simulink model "tongbukongzhi1"  (R2014b)
settings: Solver=ode45  StartTime=0.0  StopTime=10.0  RelTol=1e-3
undefined symbols (not defined in the file): sigbuilder_block
libraries: simulink x61, fuzblock x32
(part 4 of 4)

== system tongbukongzhi1/Subsystem1/Subsystem5/fuzzypid2/Subsystem ==
  In1 : Inport
  In2 : Inport  Port=2
  Add : Sum  Inputs=+++
  Demux : Demux  Outputs=3
  Derivative : Derivative
  Fuzzy Logic Controller : fuzblock/Fuzzy Logic  Controller  fis=fuzzy1
  Gain : Gain  Gain=12.9851074749726
  Gain1 : Gain  Gain=3.96505413373294
  Gain2 : Gain  Gain=0.756963167778154
  Integrator : Integrator
  Mux : Mux  Inputs=2
  Mux1 : Mux  Inputs=3
  Scope : Scope
  Sum : Sum  Inputs=|++
  Sum1 : Sum  Inputs=|++
  Sum2 : Sum  Inputs=|++
  Zero-Order Hold : ZeroOrderHold  SampleTime=0.2
  Zero-Order Hold1 : ZeroOrderHold  SampleTime=0.2
  Out1 : Outport
  wires:
  In1/1 -> Gain/1, Gain2/1, Gain1/1, Mux/1
  Derivative/1 -> Add/3
  Integrator/1 -> Add/2
  Add/1 -> Out1/1
  In2/1 -> Mux/2
  Gain/1 -> Sum2/1
  Sum2/1 -> Add/1
  Gain1/1 -> Sum1/1
  Sum1/1 -> Integrator/1
  Gain2/1 -> Sum/1
  Sum/1 -> Derivative/1
  Demux/1 -> Mux1/1, Sum2/2
  Demux/2 -> Sum1/2, Mux1/2
  Demux/3 -> Sum/2, Mux1/3
  Mux/1 -> Zero-Order Hold/1
  Fuzzy Logic Controller/1 -> Zero-Order Hold1/1
  Zero-Order Hold/1 -> Fuzzy Logic Controller/1
  Zero-Order Hold1/1 -> Demux/1
  Mux1/1 -> Scope/1

== system tongbukongzhi1/Subsystem1/Subsystem5/fuzzypid3/Subsystem ==
  In1 : Inport
  In2 : Inport  Port=2
  Add : Sum  Inputs=+++
  Demux : Demux  Outputs=3
  Derivative : Derivative
  Fuzzy Logic Controller : fuzblock/Fuzzy Logic  Controller  fis=fuzzy1
  Gain : Gain  Gain=12.9851074749726
  Gain1 : Gain  Gain=3.96505413373294
  Gain2 : Gain  Gain=0.756963167778154
  Integrator : Integrator
  Mux : Mux  Inputs=2
  Mux1 : Mux  Inputs=3
  Scope : Scope
  Sum : Sum  Inputs=|++
  Sum1 : Sum  Inputs=|++
  Sum2 : Sum  Inputs=|++
  Zero-Order Hold : ZeroOrderHold  SampleTime=0.2
  Zero-Order Hold1 : ZeroOrderHold  SampleTime=0.2
  Out1 : Outport
  wires:
  In1/1 -> Gain/1, Gain2/1, Gain1/1, Mux/1
  Derivative/1 -> Add/3
  Integrator/1 -> Add/2
  Add/1 -> Out1/1
  In2/1 -> Mux/2
  Gain/1 -> Sum2/1
  Sum2/1 -> Add/1
  Gain1/1 -> Sum1/1
  Sum1/1 -> Integrator/1
  Gain2/1 -> Sum/1
  Sum/1 -> Derivative/1
  Demux/1 -> Mux1/1, Sum2/2
  Demux/2 -> Sum1/2, Mux1/2
  Demux/3 -> Sum/2, Mux1/3
  Mux/1 -> Zero-Order Hold/1
  Fuzzy Logic Controller/1 -> Zero-Order Hold1/1
  Zero-Order Hold/1 -> Fuzzy Logic Controller/1
  Zero-Order Hold1/1 -> Demux/1
  Mux1/1 -> Scope/1

== system tongbukongzhi1/Subsystem1/Subsystem6/fuzzypid1/Subsystem ==
  In1 : Inport
  In2 : Inport  Port=2
  Add : Sum  Inputs=+++
  Demux : Demux  Outputs=3
  Derivative : Derivative
  Fuzzy Logic Controller : fuzblock/Fuzzy Logic  Controller  fis=fuzzy1
  Gain : Gain  Gain=12.9851074749726
  Gain1 : Gain  Gain=3.96505413373294
  Gain2 : Gain  Gain=0.756963167778154
  Integrator : Integrator
  Mux : Mux  Inputs=2
  Mux1 : Mux  Inputs=3
  Scope : Scope
  Sum : Sum  Inputs=|++
  Sum1 : Sum  Inputs=|++
  Sum2 : Sum  Inputs=|++
  Zero-Order Hold : ZeroOrderHold  SampleTime=0.2
  Zero-Order Hold1 : ZeroOrderHold  SampleTime=0.2
  Out1 : Outport
  wires:
  In1/1 -> Gain/1, Gain2/1, Gain1/1, Mux/1
  Derivative/1 -> Add/3
  Integrator/1 -> Add/2
  Add/1 -> Out1/1
  In2/1 -> Mux/2
  Gain/1 -> Sum2/1
  Sum2/1 -> Add/1
  Gain1/1 -> Sum1/1
  Sum1/1 -> Integrator/1
  Gain2/1 -> Sum/1
  Sum/1 -> Derivative/1
  Demux/1 -> Mux1/1, Sum2/2
  Demux/2 -> Sum1/2, Mux1/2
  Demux/3 -> Sum/2, Mux1/3
  Mux/1 -> Zero-Order Hold/1
  Fuzzy Logic Controller/1 -> Zero-Order Hold1/1
  Zero-Order Hold/1 -> Fuzzy Logic Controller/1
  Zero-Order Hold1/1 -> Demux/1
  Mux1/1 -> Scope/1

== system tongbukongzhi1/Subsystem1/Subsystem6/fuzzypid2/Subsystem ==
  In1 : Inport
  In2 : Inport  Port=2
  Add : Sum  Inputs=+++
  Demux : Demux  Outputs=3
  Derivative : Derivative
  Fuzzy Logic Controller : fuzblock/Fuzzy Logic  Controller  fis=fuzzy1
  Gain : Gain  Gain=12.9851074749726
  Gain1 : Gain  Gain=3.96505413373294
  Gain2 : Gain  Gain=0.756963167778154
  Integrator : Integrator
  Mux : Mux  Inputs=2
  Mux1 : Mux  Inputs=3
  Scope : Scope
  Sum : Sum  Inputs=|++
  Sum1 : Sum  Inputs=|++
  Sum2 : Sum  Inputs=|++
  Zero-Order Hold : ZeroOrderHold  SampleTime=0.2
  Zero-Order Hold1 : ZeroOrderHold  SampleTime=0.2
  Out1 : Outport
  wires:
  In1/1 -> Gain/1, Gain2/1, Gain1/1, Mux/1
  Derivative/1 -> Add/3
  Integrator/1 -> Add/2
  Add/1 -> Out1/1
  In2/1 -> Mux/2
  Gain/1 -> Sum2/1
  Sum2/1 -> Add/1
  Gain1/1 -> Sum1/1
  Sum1/1 -> Integrator/1
  Gain2/1 -> Sum/1
  Sum/1 -> Derivative/1
  Demux/1 -> Mux1/1, Sum2/2
  Demux/2 -> Sum1/2, Mux1/2
  Demux/3 -> Sum/2, Mux1/3
  Mux/1 -> Zero-Order Hold/1
  Fuzzy Logic Controller/1 -> Zero-Order Hold1/1
  Zero-Order Hold/1 -> Fuzzy Logic Controller/1
  Zero-Order Hold1/1 -> Demux/1
  Mux1/1 -> Scope/1

== system tongbukongzhi1/Subsystem1/Subsystem6/fuzzypid3/Subsystem ==
  In1 : Inport
  In2 : Inport  Port=2
  Add : Sum  Inputs=+++
  Demux : Demux  Outputs=3
  Derivative : Derivative
  Fuzzy Logic Controller : fuzblock/Fuzzy Logic  Controller  fis=fuzzy1
  Gain : Gain  Gain=12.9851074749726
  Gain1 : Gain  Gain=3.96505413373294
  Gain2 : Gain  Gain=0.756963167778154
  Integrator : Integrator
  Mux : Mux  Inputs=2
  Mux1 : Mux  Inputs=3
  Scope : Scope
  Sum : Sum  Inputs=|++
  Sum1 : Sum  Inputs=|++
  Sum2 : Sum  Inputs=|++
  Zero-Order Hold : ZeroOrderHold  SampleTime=0.2
  Zero-Order Hold1 : ZeroOrderHold  SampleTime=0.2
  Out1 : Outport
  wires:
  In1/1 -> Gain/1, Gain2/1, Gain1/1, Mux/1
  Derivative/1 -> Add/3
  Integrator/1 -> Add/2
  Add/1 -> Out1/1
  In2/1 -> Mux/2
  Gain/1 -> Sum2/1
  Sum2/1 -> Add/1
  Gain1/1 -> Sum1/1
  Sum1/1 -> Integrator/1
  Gain2/1 -> Sum/1
  Sum/1 -> Derivative/1
  Demux/1 -> Mux1/1, Sum2/2
  Demux/2 -> Sum1/2, Mux1/2
  Demux/3 -> Sum/2, Mux1/3
  Mux/1 -> Zero-Order Hold/1
  Fuzzy Logic Controller/1 -> Zero-Order Hold1/1
  Zero-Order Hold/1 -> Fuzzy Logic Controller/1
  Zero-Order Hold1/1 -> Demux/1
  Mux1/1 -> Scope/1

== system tongbukongzhi1/Subsystem1/Subsystem7/fuzzypid1/Subsystem ==
  In1 : Inport
  In2 : Inport  Port=2
  Add : Sum  Inputs=+++
  Demux : Demux  Outputs=3
  Derivative : Derivative
  Fuzzy Logic Controller : fuzblock/Fuzzy Logic  Controller  fis=fuzzy1
  Gain : Gain  Gain=12.9851074749726
  Gain1 : Gain  Gain=3.96505413373294
  Gain2 : Gain  Gain=0.756963167778154
  Integrator : Integrator
  Mux : Mux  Inputs=2
  Mux1 : Mux  Inputs=3
  Scope : Scope
  Sum : Sum  Inputs=|++
  Sum1 : Sum  Inputs=|++
  Sum2 : Sum  Inputs=|++
  Zero-Order Hold : ZeroOrderHold  SampleTime=0.2
  Zero-Order Hold1 : ZeroOrderHold  SampleTime=0.2
  Out1 : Outport
  wires:
  In1/1 -> Gain/1, Gain2/1, Gain1/1, Mux/1
  Derivative/1 -> Add/3
  Integrator/1 -> Add/2
  Add/1 -> Out1/1
  In2/1 -> Mux/2
  Gain/1 -> Sum2/1
  Sum2/1 -> Add/1
  Gain1/1 -> Sum1/1
  Sum1/1 -> Integrator/1
  Gain2/1 -> Sum/1
  Sum/1 -> Derivative/1
  Demux/1 -> Mux1/1, Sum2/2
  Demux/2 -> Sum1/2, Mux1/2
  Demux/3 -> Sum/2, Mux1/3
  Mux/1 -> Zero-Order Hold/1
  Fuzzy Logic Controller/1 -> Zero-Order Hold1/1
  Zero-Order Hold/1 -> Fuzzy Logic Controller/1
  Zero-Order Hold1/1 -> Demux/1
  Mux1/1 -> Scope/1

== system tongbukongzhi1/Subsystem1/Subsystem7/fuzzypid2/Subsystem ==
  In1 : Inport
  In2 : Inport  Port=2
  Add : Sum  Inputs=+++
  Demux : Demux  Outputs=3
  Derivative : Derivative
  Fuzzy Logic Controller : fuzblock/Fuzzy Logic  Controller  fis=fuzzy1
  Gain : Gain  Gain=12.9851074749726
  Gain1 : Gain  Gain=3.96505413373294
  Gain2 : Gain  Gain=0.756963167778154
  Integrator : Integrator
  Mux : Mux  Inputs=2
  Mux1 : Mux  Inputs=3
  Scope : Scope
  Sum : Sum  Inputs=|++
  Sum1 : Sum  Inputs=|++
  Sum2 : Sum  Inputs=|++
  Zero-Order Hold : ZeroOrderHold  SampleTime=0.2
  Zero-Order Hold1 : ZeroOrderHold  SampleTime=0.2
  Out1 : Outport
  wires:
  In1/1 -> Gain/1, Gain2/1, Gain1/1, Mux/1
  Derivative/1 -> Add/3
  Integrator/1 -> Add/2
  Add/1 -> Out1/1
  In2/1 -> Mux/2
  Gain/1 -> Sum2/1
  Sum2/1 -> Add/1
  Gain1/1 -> Sum1/1
  Sum1/1 -> Integrator/1
  Gain2/1 -> Sum/1
  Sum/1 -> Derivative/1
  Demux/1 -> Mux1/1, Sum2/2
  Demux/2 -> Sum1/2, Mux1/2
  Demux/3 -> Sum/2, Mux1/3
  Mux/1 -> Zero-Order Hold/1
  Fuzzy Logic Controller/1 -> Zero-Order Hold1/1
  Zero-Order Hold/1 -> Fuzzy Logic Controller/1
  Zero-Order Hold1/1 -> Demux/1
  Mux1/1 -> Scope/1

== system tongbukongzhi1/Subsystem1/Subsystem7/fuzzypid3/Subsystem ==
  In1 : Inport
  In2 : Inport  Port=2
  Add : Sum  Inputs=+++
  Demux : Demux  Outputs=3
  Derivative : Derivative
  Fuzzy Logic Controller : fuzblock/Fuzzy Logic  Controller  fis=fuzzy1
  Gain : Gain  Gain=12.9851074749726
  Gain1 : Gain  Gain=3.96505413373294
  Gain2 : Gain  Gain=0.756963167778154
  Integrator : Integrator
  Mux : Mux  Inputs=2
  Mux1 : Mux  Inputs=3
  Scope : Scope
  Sum : Sum  Inputs=|++
  Sum1 : Sum  Inputs=|++
  Sum2 : Sum  Inputs=|++
  Zero-Order Hold : ZeroOrderHold  SampleTime=0.2
  Zero-Order Hold1 : ZeroOrderHold  SampleTime=0.2
  Out1 : Outport
  wires:
  In1/1 -> Gain/1, Gain2/1, Gain1/1, Mux/1
  Derivative/1 -> Add/3
  Integrator/1 -> Add/2
  Add/1 -> Out1/1
  In2/1 -> Mux/2
  Gain/1 -> Sum2/1
  Sum2/1 -> Add/1
  Gain1/1 -> Sum1/1
  Sum1/1 -> Integrator/1
  Gain2/1 -> Sum/1
  Sum/1 -> Derivative/1
  Demux/1 -> Mux1/1, Sum2/2
  Demux/2 -> Sum1/2, Mux1/2
  Demux/3 -> Sum/2, Mux1/3
  Mux/1 -> Zero-Order Hold/1
  Fuzzy Logic Controller/1 -> Zero-Order Hold1/1
  Zero-Order Hold/1 -> Fuzzy Logic Controller/1
  Zero-Order Hold1/1 -> Demux/1
  Mux1/1 -> Scope/1

== system tongbukongzhi1/Subsystem4/Subsystem/fuzzypid1/Subsystem ==
  In1 : Inport
  In2 : Inport  Port=2
  Add : Sum  Inputs=+++
  Demux : Demux  Outputs=3
  Derivative : Derivative
  Fuzzy Logic Controller : fuzblock/Fuzzy Logic  Controller  fis=fuzzy1
  Gain : Gain  Gain=12.9851074749726
  Gain1 : Gain  Gain=3.96505413373294
  Gain2 : Gain  Gain=0.756963167778154
  Integrator : Integrator
  Mux : Mux  Inputs=2
  Mux1 : Mux  Inputs=3
  Scope : Scope
      settings: YMin=-0.2  YMax=0.05
  Sum : Sum  Inputs=|++
  Sum1 : Sum  Inputs=|++
  Sum2 : Sum  Inputs=|++
  Zero-Order Hold : ZeroOrderHold  SampleTime=0.1
  Zero-Order Hold1 : ZeroOrderHold  SampleTime=0.1
  Out1 : Outport
  wires:
  In1/1 -> Gain/1, Gain2/1, Gain1/1, Mux/1
  Derivative/1 -> Add/3
  Integrator/1 -> Add/2
  Add/1 -> Out1/1
  In2/1 -> Mux/2
  Gain/1 -> Sum2/1
  Sum2/1 -> Add/1
  Gain1/1 -> Sum1/1
  Sum1/1 -> Integrator/1
  Gain2/1 -> Sum/1
  Sum/1 -> Derivative/1
  Mux/1 -> Zero-Order Hold/1
  Fuzzy Logic Controller/1 -> Zero-Order Hold1/1
  Zero-Order Hold/1 -> Fuzzy Logic Controller/1
  Zero-Order Hold1/1 -> Demux/1
  Mux1/1 -> Scope/1
  Demux/3 -> Sum/2, Mux1/3
  Demux/2 -> Sum1/2, Mux1/2
  Demux/1 -> Mux1/1, Sum2/2

== system tongbukongzhi1/Subsystem4/Subsystem/fuzzypid2/Subsystem ==
  In1 : Inport
  In2 : Inport  Port=2
  Add : Sum  Inputs=+++
  Demux : Demux  Outputs=3
  Derivative : Derivative
  Fuzzy Logic Controller : fuzblock/Fuzzy Logic  Controller  fis=fuzzy1
  Gain : Gain  Gain=12.9851074749726
  Gain1 : Gain  Gain=3.96505413373294
  Gain2 : Gain  Gain=0.756963167778154
  Integrator : Integrator
  Mux : Mux  Inputs=2
  Mux1 : Mux  Inputs=3
  Scope : Scope
      settings: YMin=-0.2  YMax=0.05
  Sum : Sum  Inputs=|++
  Sum1 : Sum  Inputs=|++
  Sum2 : Sum  Inputs=|++
  Zero-Order Hold : ZeroOrderHold  SampleTime=0.1
  Zero-Order Hold1 : ZeroOrderHold  SampleTime=0.1
  Out1 : Outport
  wires:
  In1/1 -> Gain/1, Gain2/1, Gain1/1, Mux/1
  Derivative/1 -> Add/3
  Integrator/1 -> Add/2
  Add/1 -> Out1/1
  In2/1 -> Mux/2
  Gain/1 -> Sum2/1
  Sum2/1 -> Add/1
  Gain1/1 -> Sum1/1
  Sum1/1 -> Integrator/1
  Gain2/1 -> Sum/1
  Sum/1 -> Derivative/1
  Mux/1 -> Zero-Order Hold/1
  Fuzzy Logic Controller/1 -> Zero-Order Hold1/1
  Zero-Order Hold/1 -> Fuzzy Logic Controller/1
  Zero-Order Hold1/1 -> Demux/1
  Mux1/1 -> Scope/1
  Demux/3 -> Sum/2, Mux1/3
  Demux/2 -> Sum1/2, Mux1/2
  Demux/1 -> Mux1/1, Sum2/2

== system tongbukongzhi1/Subsystem4/Subsystem/fuzzypid4/Subsystem ==
  In1 : Inport
  In2 : Inport  Port=2
  Add : Sum  Inputs=+++
  Demux : Demux  Outputs=3
  Derivative : Derivative
  Fuzzy Logic Controller : fuzblock/Fuzzy Logic  Controller  fis=fuzzy1
  Gain : Gain  Gain=12.9851074749726
  Gain1 : Gain  Gain=3.96505413373294
  Gain2 : Gain  Gain=0.756963167778154
  Integrator : Integrator
  Mux : Mux  Inputs=2
  Mux1 : Mux  Inputs=3
  Scope : Scope
      settings: YMin=-0.2  YMax=0.05
  Sum : Sum  Inputs=|++
  Sum1 : Sum  Inputs=|++
  Sum2 : Sum  Inputs=|++
  Zero-Order Hold : ZeroOrderHold  SampleTime=0.1
  Zero-Order Hold1 : ZeroOrderHold  SampleTime=0.1
  Out1 : Outport
  wires:
  In1/1 -> Gain/1, Gain2/1, Gain1/1, Mux/1
  Derivative/1 -> Add/3
  Integrator/1 -> Add/2
  Add/1 -> Out1/1
  In2/1 -> Mux/2
  Gain/1 -> Sum2/1
  Sum2/1 -> Add/1
  Gain1/1 -> Sum1/1
  Sum1/1 -> Integrator/1
  Gain2/1 -> Sum/1
  Sum/1 -> Derivative/1
  Mux/1 -> Zero-Order Hold/1
  Fuzzy Logic Controller/1 -> Zero-Order Hold1/1
  Zero-Order Hold/1 -> Fuzzy Logic Controller/1
  Zero-Order Hold1/1 -> Demux/1
  Mux1/1 -> Scope/1
  Demux/3 -> Sum/2, Mux1/3
  Demux/2 -> Sum1/2, Mux1/2
  Demux/1 -> Mux1/1, Sum2/2

== system tongbukongzhi1/Subsystem4/Subsystem1/fuzzypid4/Subsystem ==
  In1 : Inport
  In2 : Inport  Port=2
  Add : Sum  Inputs=+++
  Demux : Demux  Outputs=3
  Derivative : Derivative
  Fuzzy Logic Controller : fuzblock/Fuzzy Logic  Controller  fis=fuzzy1
  Gain : Gain  Gain=12.9851074749726
  Gain1 : Gain  Gain=3.96505413373294
  Gain2 : Gain  Gain=0.756963167778154
  Integrator : Integrator
  Mux : Mux  Inputs=2
  Mux1 : Mux  Inputs=3
  Scope : Scope
      settings: YMin=-0.2  YMax=0.05
  Sum : Sum  Inputs=|++
  Sum1 : Sum  Inputs=|++
  Sum2 : Sum  Inputs=|++
  Zero-Order Hold : ZeroOrderHold  SampleTime=0.1
  Zero-Order Hold1 : ZeroOrderHold  SampleTime=0.1
  Out1 : Outport
  wires:
  In1/1 -> Gain/1, Gain2/1, Gain1/1, Mux/1
  Derivative/1 -> Add/3
  Integrator/1 -> Add/2
  Add/1 -> Out1/1
  In2/1 -> Mux/2
  Gain/1 -> Sum2/1
  Sum2/1 -> Add/1
  Gain1/1 -> Sum1/1
  Sum1/1 -> Integrator/1
  Gain2/1 -> Sum/1
  Sum/1 -> Derivative/1
  Mux/1 -> Zero-Order Hold/1
  Fuzzy Logic Controller/1 -> Zero-Order Hold1/1
  Zero-Order Hold/1 -> Fuzzy Logic Controller/1
  Zero-Order Hold1/1 -> Demux/1
  Mux1/1 -> Scope/1
  Demux/3 -> Sum/2, Mux1/3
  Demux/2 -> Sum1/2, Mux1/2
  Demux/1 -> Mux1/1, Sum2/2

== system tongbukongzhi1/Subsystem4/Subsystem1/fuzzypid5/Subsystem ==
  In1 : Inport
  In2 : Inport  Port=2
  Add : Sum  Inputs=+++
  Demux : Demux  Outputs=3
  Derivative : Derivative
  Fuzzy Logic Controller : fuzblock/Fuzzy Logic  Controller  fis=fuzzy1
  Gain : Gain  Gain=12.9851074749726
  Gain1 : Gain  Gain=3.96505413373294
  Gain2 : Gain  Gain=0.756963167778154
  Integrator : Integrator
  Mux : Mux  Inputs=2
  Mux1 : Mux  Inputs=3
  Scope : Scope
      settings: YMin=-0.2  YMax=0.05
  Sum : Sum  Inputs=|++
  Sum1 : Sum  Inputs=|++
  Sum2 : Sum  Inputs=|++
  Zero-Order Hold : ZeroOrderHold  SampleTime=0.1
  Zero-Order Hold1 : ZeroOrderHold  SampleTime=0.1
  Out1 : Outport
  wires:
  In1/1 -> Gain/1, Gain2/1, Gain1/1, Mux/1
  Derivative/1 -> Add/3
  Integrator/1 -> Add/2
  Add/1 -> Out1/1
  In2/1 -> Mux/2
  Gain/1 -> Sum2/1
  Sum2/1 -> Add/1
  Gain1/1 -> Sum1/1
  Sum1/1 -> Integrator/1
  Gain2/1 -> Sum/1
  Sum/1 -> Derivative/1
  Mux/1 -> Zero-Order Hold/1
  Fuzzy Logic Controller/1 -> Zero-Order Hold1/1
  Zero-Order Hold/1 -> Fuzzy Logic Controller/1
  Zero-Order Hold1/1 -> Demux/1
  Mux1/1 -> Scope/1
  Demux/3 -> Sum/2, Mux1/3
  Demux/2 -> Sum1/2, Mux1/2
  Demux/1 -> Mux1/1, Sum2/2

== system tongbukongzhi1/Subsystem4/Subsystem1/fuzzypid6/Subsystem ==
  In1 : Inport
  In2 : Inport  Port=2
  Add : Sum  Inputs=+++
  Demux : Demux  Outputs=3
  Derivative : Derivative
  Fuzzy Logic Controller : fuzblock/Fuzzy Logic  Controller  fis=fuzzy1
  Gain : Gain  Gain=12.9851074749726
  Gain1 : Gain  Gain=3.96505413373294
  Gain2 : Gain  Gain=0.756963167778154
  Integrator : Integrator
  Mux : Mux  Inputs=2
  Mux1 : Mux  Inputs=3
  Scope : Scope
      settings: YMin=-0.2  YMax=0.05
  Sum : Sum  Inputs=|++
  Sum1 : Sum  Inputs=|++
  Sum2 : Sum  Inputs=|++
  Zero-Order Hold : ZeroOrderHold  SampleTime=0.1
  Zero-Order Hold1 : ZeroOrderHold  SampleTime=0.1
  Out1 : Outport
  wires:
  In1/1 -> Gain/1, Gain2/1, Gain1/1, Mux/1
  Derivative/1 -> Add/3
  Integrator/1 -> Add/2
  Add/1 -> Out1/1
  In2/1 -> Mux/2
  Gain/1 -> Sum2/1
  Sum2/1 -> Add/1
  Gain1/1 -> Sum1/1
  Sum1/1 -> Integrator/1
  Gain2/1 -> Sum/1
  Sum/1 -> Derivative/1
  Mux/1 -> Zero-Order Hold/1
  Fuzzy Logic Controller/1 -> Zero-Order Hold1/1
  Zero-Order Hold/1 -> Fuzzy Logic Controller/1
  Zero-Order Hold1/1 -> Demux/1
  Mux1/1 -> Scope/1
  Demux/3 -> Sum/2, Mux1/3
  Demux/2 -> Sum1/2, Mux1/2
  Demux/1 -> Mux1/1, Sum2/2

== system tongbukongzhi1/Subsystem4/Subsystem2/fuzzypid4/Subsystem ==
  In1 : Inport
  In2 : Inport  Port=2
  Add : Sum  Inputs=+++
  Demux : Demux  Outputs=3
  Derivative : Derivative
  Fuzzy Logic Controller : fuzblock/Fuzzy Logic  Controller  fis=fuzzy1
  Gain : Gain  Gain=12.9851074749726
  Gain1 : Gain  Gain=3.96505413373294
  Gain2 : Gain  Gain=0.756963167778154
  Integrator : Integrator
  Mux : Mux  Inputs=2
  Mux1 : Mux  Inputs=3
  Scope : Scope
      settings: YMin=-0.2  YMax=0.05
  Sum : Sum  Inputs=|++
  Sum1 : Sum  Inputs=|++
  Sum2 : Sum  Inputs=|++
  Zero-Order Hold : ZeroOrderHold  SampleTime=0.1
  Zero-Order Hold1 : ZeroOrderHold  SampleTime=0.1
  Out1 : Outport
  wires:
  In1/1 -> Gain/1, Gain2/1, Gain1/1, Mux/1
  Derivative/1 -> Add/3
  Integrator/1 -> Add/2
  Add/1 -> Out1/1
  In2/1 -> Mux/2
  Gain/1 -> Sum2/1
  Sum2/1 -> Add/1
  Gain1/1 -> Sum1/1
  Sum1/1 -> Integrator/1
  Gain2/1 -> Sum/1
  Sum/1 -> Derivative/1
  Mux/1 -> Zero-Order Hold/1
  Fuzzy Logic Controller/1 -> Zero-Order Hold1/1
  Zero-Order Hold/1 -> Fuzzy Logic Controller/1
  Zero-Order Hold1/1 -> Demux/1
  Mux1/1 -> Scope/1
  Demux/3 -> Sum/2, Mux1/3
  Demux/2 -> Sum1/2, Mux1/2
  Demux/1 -> Mux1/1, Sum2/2

== system tongbukongzhi1/Subsystem4/Subsystem2/fuzzypid5/Subsystem ==
  In1 : Inport
  In2 : Inport  Port=2
  Add : Sum  Inputs=+++
  Demux : Demux  Outputs=3
  Derivative : Derivative
  Fuzzy Logic Controller : fuzblock/Fuzzy Logic  Controller  fis=fuzzy1
  Gain : Gain  Gain=12.9851074749726
  Gain1 : Gain  Gain=3.96505413373294
  Gain2 : Gain  Gain=0.756963167778154
  Integrator : Integrator
  Mux : Mux  Inputs=2
  Mux1 : Mux  Inputs=3
  Scope : Scope
      settings: YMin=-0.2  YMax=0.05
  Sum : Sum  Inputs=|++
  Sum1 : Sum  Inputs=|++
  Sum2 : Sum  Inputs=|++
  Zero-Order Hold : ZeroOrderHold  SampleTime=0.1
  Zero-Order Hold1 : ZeroOrderHold  SampleTime=0.1
  Out1 : Outport
  wires:
  In1/1 -> Gain/1, Gain2/1, Gain1/1, Mux/1
  Derivative/1 -> Add/3
  Integrator/1 -> Add/2
  Add/1 -> Out1/1
  In2/1 -> Mux/2
  Gain/1 -> Sum2/1
  Sum2/1 -> Add/1
  Gain1/1 -> Sum1/1
  Sum1/1 -> Integrator/1
  Gain2/1 -> Sum/1
  Sum/1 -> Derivative/1
  Mux/1 -> Zero-Order Hold/1
  Fuzzy Logic Controller/1 -> Zero-Order Hold1/1
  Zero-Order Hold/1 -> Fuzzy Logic Controller/1
  Zero-Order Hold1/1 -> Demux/1
  Mux1/1 -> Scope/1
  Demux/3 -> Sum/2, Mux1/3
  Demux/2 -> Sum1/2, Mux1/2
  Demux/1 -> Mux1/1, Sum2/2

== system tongbukongzhi1/Subsystem4/Subsystem2/fuzzypid6/Subsystem ==
  In1 : Inport
  In2 : Inport  Port=2
  Add : Sum  Inputs=+++
  Demux : Demux  Outputs=3
  Derivative : Derivative
  Fuzzy Logic Controller : fuzblock/Fuzzy Logic  Controller  fis=fuzzy1
  Gain : Gain  Gain=12.9851074749726
  Gain1 : Gain  Gain=3.96505413373294
  Gain2 : Gain  Gain=0.756963167778154
  Integrator : Integrator
  Mux : Mux  Inputs=2
  Mux1 : Mux  Inputs=3
  Scope : Scope
      settings: YMin=-0.2  YMax=0.05
  Sum : Sum  Inputs=|++
  Sum1 : Sum  Inputs=|++
  Sum2 : Sum  Inputs=|++
  Zero-Order Hold : ZeroOrderHold  SampleTime=0.1
  Zero-Order Hold1 : ZeroOrderHold  SampleTime=0.1
  Out1 : Outport
  wires:
  In1/1 -> Gain/1, Gain2/1, Gain1/1, Mux/1
  Derivative/1 -> Add/3
  Integrator/1 -> Add/2
  Add/1 -> Out1/1
  In2/1 -> Mux/2
  Gain/1 -> Sum2/1
  Sum2/1 -> Add/1
  Gain1/1 -> Sum1/1
  Sum1/1 -> Integrator/1
  Gain2/1 -> Sum/1
  Sum/1 -> Derivative/1
  Mux/1 -> Zero-Order Hold/1
  Fuzzy Logic Controller/1 -> Zero-Order Hold1/1
  Zero-Order Hold/1 -> Fuzzy Logic Controller/1
  Zero-Order Hold1/1 -> Demux/1
  Mux1/1 -> Scope/1
  Demux/3 -> Sum/2, Mux1/3
  Demux/2 -> Sum1/2, Mux1/2
  Demux/1 -> Mux1/1, Sum2/2

== system tongbukongzhi1/Subsystem4/Subsystem3/fuzzypid4/Subsystem ==
  In1 : Inport
  In2 : Inport  Port=2
  Add : Sum  Inputs=+++
  Demux : Demux  Outputs=3
  Derivative : Derivative
  Fuzzy Logic Controller : fuzblock/Fuzzy Logic  Controller  fis=fuzzy1
  Gain : Gain  Gain=12.9851074749726
  Gain1 : Gain  Gain=3.96505413373294
  Gain2 : Gain  Gain=0.756963167778154
  Integrator : Integrator
  Mux : Mux  Inputs=2
  Mux1 : Mux  Inputs=3
  Scope : Scope
      settings: YMin=-0.2  YMax=0.05
  Sum : Sum  Inputs=|++
  Sum1 : Sum  Inputs=|++
  Sum2 : Sum  Inputs=|++
  Zero-Order Hold : ZeroOrderHold  SampleTime=0.1
  Zero-Order Hold1 : ZeroOrderHold  SampleTime=0.1
  Out1 : Outport
  wires:
  In1/1 -> Gain/1, Gain2/1, Gain1/1, Mux/1
  Derivative/1 -> Add/3
  Integrator/1 -> Add/2
  Add/1 -> Out1/1
  In2/1 -> Mux/2
  Gain/1 -> Sum2/1
  Sum2/1 -> Add/1
  Gain1/1 -> Sum1/1
  Sum1/1 -> Integrator/1
  Gain2/1 -> Sum/1
  Sum/1 -> Derivative/1
  Mux/1 -> Zero-Order Hold/1
  Fuzzy Logic Controller/1 -> Zero-Order Hold1/1
  Zero-Order Hold/1 -> Fuzzy Logic Controller/1
  Zero-Order Hold1/1 -> Demux/1
  Mux1/1 -> Scope/1
  Demux/3 -> Sum/2, Mux1/3
  Demux/2 -> Sum1/2, Mux1/2
  Demux/1 -> Mux1/1, Sum2/2

== system tongbukongzhi1/Subsystem4/Subsystem3/fuzzypid5/Subsystem ==
  In1 : Inport
  In2 : Inport  Port=2
  Add : Sum  Inputs=+++
  Demux : Demux  Outputs=3
  Derivative : Derivative
  Fuzzy Logic Controller : fuzblock/Fuzzy Logic  Controller  fis=fuzzy1
  Gain : Gain  Gain=12.9851074749726
  Gain1 : Gain  Gain=3.96505413373294
  Gain2 : Gain  Gain=0.756963167778154
  Integrator : Integrator
  Mux : Mux  Inputs=2
  Mux1 : Mux  Inputs=3
  Scope : Scope
      settings: YMin=-0.2  YMax=0.05
  Sum : Sum  Inputs=|++
  Sum1 : Sum  Inputs=|++
  Sum2 : Sum  Inputs=|++
  Zero-Order Hold : ZeroOrderHold  SampleTime=0.1
  Zero-Order Hold1 : ZeroOrderHold  SampleTime=0.1
  Out1 : Outport
  wires:
  In1/1 -> Gain/1, Gain2/1, Gain1/1, Mux/1
  Derivative/1 -> Add/3
  Integrator/1 -> Add/2
  Add/1 -> Out1/1
  In2/1 -> Mux/2
  Gain/1 -> Sum2/1
  Sum2/1 -> Add/1
  Gain1/1 -> Sum1/1
  Sum1/1 -> Integrator/1
  Gain2/1 -> Sum/1
  Sum/1 -> Derivative/1
  Mux/1 -> Zero-Order Hold/1
  Fuzzy Logic Controller/1 -> Zero-Order Hold1/1
  Zero-Order Hold/1 -> Fuzzy Logic Controller/1
  Zero-Order Hold1/1 -> Demux/1
  Mux1/1 -> Scope/1
  Demux/3 -> Sum/2, Mux1/3
  Demux/2 -> Sum1/2, Mux1/2
  Demux/1 -> Mux1/1, Sum2/2

== system tongbukongzhi1/Subsystem4/Subsystem3/fuzzypid6/Subsystem ==
  In1 : Inport
  In2 : Inport  Port=2
  Add : Sum  Inputs=+++
  Demux : Demux  Outputs=3
  Derivative : Derivative
  Fuzzy Logic Controller : fuzblock/Fuzzy Logic  Controller  fis=fuzzy1
  Gain : Gain  Gain=12.9851074749726
  Gain1 : Gain  Gain=3.96505413373294
  Gain2 : Gain  Gain=0.756963167778154
  Integrator : Integrator
  Mux : Mux  Inputs=2
  Mux1 : Mux  Inputs=3
  Scope : Scope
      settings: YMin=-0.2  YMax=0.05
  Sum : Sum  Inputs=|++
  Sum1 : Sum  Inputs=|++
  Sum2 : Sum  Inputs=|++
  Zero-Order Hold : ZeroOrderHold  SampleTime=0.1
  Zero-Order Hold1 : ZeroOrderHold  SampleTime=0.1
  Out1 : Outport
  wires:
  In1/1 -> Gain/1, Gain2/1, Gain1/1, Mux/1
  Derivative/1 -> Add/3
  Integrator/1 -> Add/2
  Add/1 -> Out1/1
  In2/1 -> Mux/2
  Gain/1 -> Sum2/1
  Sum2/1 -> Add/1
  Gain1/1 -> Sum1/1
  Sum1/1 -> Integrator/1
  Gain2/1 -> Sum/1
  Sum/1 -> Derivative/1
  Mux/1 -> Zero-Order Hold/1
  Fuzzy Logic Controller/1 -> Zero-Order Hold1/1
  Zero-Order Hold/1 -> Fuzzy Logic Controller/1
  Zero-Order Hold1/1 -> Demux/1
  Mux1/1 -> Scope/1
  Demux/3 -> Sum/2, Mux1/3
  Demux/2 -> Sum1/2, Mux1/2
  Demux/1 -> Mux1/1, Sum2/2
